simulink model "experimento2_sim"  (R2014a)
settings: Solver=ode45  StartTime=0.0  StopTime=5  RelTol=1e-3
values from neighbouring files (symbols this model uses):
  a = [-1 -1; 6.5 0]    [experimento2_01.m]
  b = [1 1; 0 1]    [experimento2_01.m]
  k = place(a,b,P1)    [experimento2_01.m]
  k1 = place(a,b,P2)    [experimento2_01.m]
  k2 = place(a,b,P3)    [experimento2_01.m]
settings Model: Creator=unieerisantos  LastModifiedBy=unieerisantos

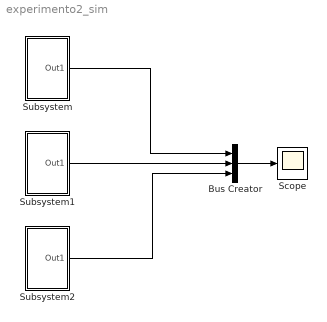
== system experimento2_sim ==
  Bus Creator : BusCreator  Inputs=3
  Scope : Scope
  Subsystem : Subsystem
  Subsystem1 : Subsystem
  Subsystem2 : Subsystem
  wires:
  Bus Creator/1 -> Scope/1
  Subsystem/1(Out1) -> Bus Creator/1
  Subsystem1/1(Out1) -> Bus Creator/2
  Subsystem2/1(Out1) -> Bus Creator/3

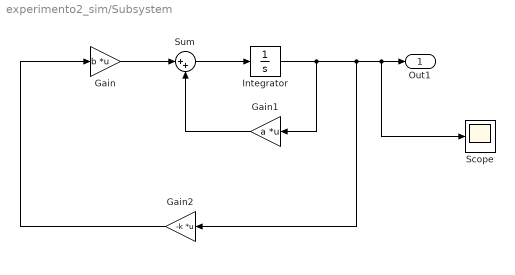
== system experimento2_sim/Subsystem ==
  Gain : Gain  Gain=b  Multiplication=Matrix(K*u)
  Gain1 : Gain  Gain=a  Multiplication=Matrix(K*u)
  Gain2 : Gain  Gain=-k  Multiplication=Matrix(K*u)
  Integrator : Integrator  InitialCondition=[+1 +5]
  Scope : Scope
  Sum : Sum  Inputs=|++
  Out1 : Outport
  wires:
  Gain/1 -> Sum/1
  Gain1/1 -> Sum/2
  Gain2/1 -> Gain/1
  Integrator/1 -> Gain1/1, Scope/1, Out1/1, Gain2/1
  Sum/1 -> Integrator/1

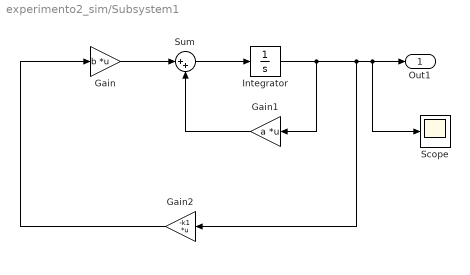
== system experimento2_sim/Subsystem1 ==
  Gain : Gain  Gain=b  Multiplication=Matrix(K*u)
  Gain1 : Gain  Gain=a  Multiplication=Matrix(K*u)
  Gain2 : Gain  Gain=-k1  Multiplication=Matrix(K*u)
  Integrator : Integrator  InitialCondition=[+1 +5]
  Scope : Scope
      settings: SaveName=ScopeData2
  Sum : Sum  Inputs=|++
  Out1 : Outport
  wires:
  Gain/1 -> Sum/1
  Gain1/1 -> Sum/2
  Gain2/1 -> Gain/1
  Integrator/1 -> Gain1/1, Scope/1, Out1/1, Gain2/1
  Sum/1 -> Integrator/1

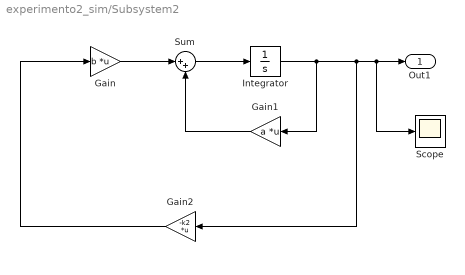
== system experimento2_sim/Subsystem2 ==
  Gain : Gain  Gain=b  Multiplication=Matrix(K*u)
  Gain1 : Gain  Gain=a  Multiplication=Matrix(K*u)
  Gain2 : Gain  Gain=-k2  Multiplication=Matrix(K*u)
  Integrator : Integrator  InitialCondition=[+1 +5]
  Scope : Scope
      settings: SaveName=ScopeData3
  Sum : Sum  Inputs=|++
  Out1 : Outport
  wires:
  Gain/1 -> Sum/1
  Gain1/1 -> Sum/2
  Gain2/1 -> Gain/1
  Integrator/1 -> Gain1/1, Scope/1, Out1/1, Gain2/1
  Sum/1 -> Integrator/1
